simulink model "LgrstOpenLStateCtrl"  (R2018b)
settings: Solver=FixedStepDiscrete  StartTime=0.0  StopTime=10.0  FixedStep=0.01  RelTol=1e-3
libraries: StateCtrlLib x1
settings Model: Creator=sn2xws  LastModifiedBy=sn2xws
settings DataIOCC: SaveFormat=StructureWithTime
settings OptimizationCC: DefaultParameterBehavior=Inlined  EnhancedBackFolding=on  PassReuseOutputArgsAs=Individual arguments  ZeroExternalMemoryAtStartup=off  ZeroInternalMemoryAtStartup=off  OptimizeBlockOrder=speed  DifferentSizesBufferReuse=on  OptimizationCustomize=off
settings DebuggingCC: ParameterTunabilityLossMsg=error
settings ModelReferenceCC: ModelReferenceNumInstancesAllowed=Single
settings SFSimCC: MATLABDynamicMemAlloc=off
settings RTWCC: SystemTargetFile=autosar.tlc  GenCodeOnly=on  TemplateMakefile=ert_default_tmf  Description=AUTOSAR  GenerateReport=on  IncludeHyperlinkInReport=on  LaunchReport=on  GenerateTraceInfo=on  GenerateTraceReport=on  GenerateTraceReportSl=on  GenerateTraceReportSf=on  GenerateTraceReportEml=on
settings CodeAppCC: ForceParamTrailComments=on  IgnoreCustomStorageClasses=off  OperatorAnnotations=on  SimulinkDataObjDesc=on  SFDataObjDesc=on  InsertBlockDesc=on
settings STFCustomTargetCC: TargetLangStandard=C99 (ISO)  MultiwordLength=256  ParMdlRefBuildCompliant=on  CompOptLevelCompliant=on  IncludeMdlTerminateFcn=off  CombineOutputUpdateFcns=on  SuppressErrorStatus=on  ERTCustomFileBanners=on  SupportNonFinite=off  SupportComplex=off  SupportContinuousTime=off  SupportNonInlinedSFcns=off  RemoveResetFunc=on  MATLABClassNameForMDSCustomization=Simulink.SoftwareTarget.ERTCustomization  AutosarCompliant=on  UseToolchainInfoCompliant=on  LookupTableObjectStructAxisOrder=2,1,3,4,...  LUTObjectStructOrderEvenSpacing=Size,Table,Breakpoints  SystemTargetFile=autosar.tlc
settings ERTTargetCC: TargetLangStandard=C99 (ISO)  ConcurrentExecutionCompliant=off  IncludeMdlTerminateFcn=off  SuppressErrorStatus=on  SupportNonFinite=off  SupportComplex=off  ModelStepFunctionPrototypeControlCompliant=off  CPPClassGenCompliant=off  AutosarCompliant=on  LookupTableObjectStructAxisOrder=2,1,3,4,...  LUTObjectStructOrderEvenSpacing=Size,Table,Breakpoints  InlinedParameterPlacement=NonHierarchical  ERTCustomFileTemplate=example_file_process.tlc

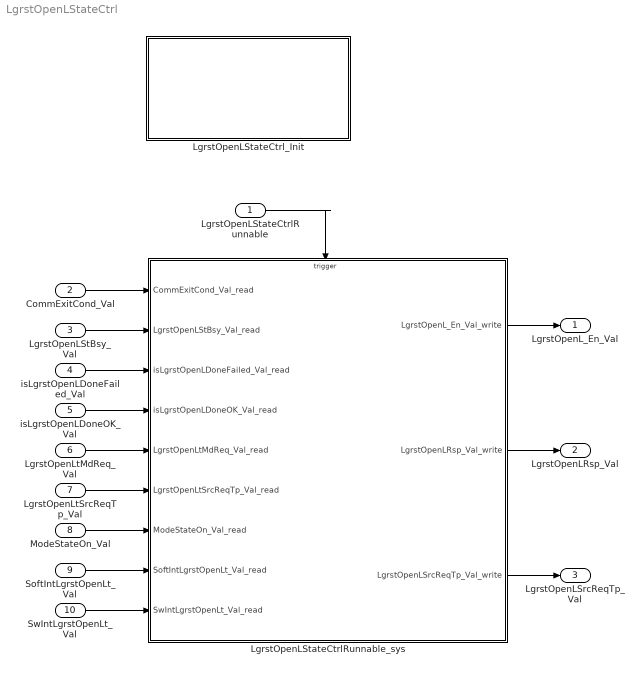
== system LgrstOpenLStateCtrl ==
  LgrstOpenLStateCtrlRunnable : Inport  SampleTime=0.01  OutputFunctionCall=on
  CommExitCond_Val : Inport  Port=2  OutDataTypeStr=boolean  PortDimensions=1
  LgrstOpenLStBsy_Val : Inport  Port=3  OutDataTypeStr=boolean  PortDimensions=1
  isLgrstOpenLDoneFailed_Val : Inport  Port=4  OutDataTypeStr=boolean  PortDimensions=1
  isLgrstOpenLDoneOK_Val : Inport  Port=5  OutDataTypeStr=boolean  PortDimensions=1
  LgrstOpenLtMdReq_Val : Inport  Port=6  OutDataTypeStr=boolean  PortDimensions=1
  LgrstOpenLtSrcReqTp_Val : Inport  Port=7  OutDataTypeStr=Enum: SrcReqTp1  PortDimensions=1
  ModeStateOn_Val : Inport  Port=8  OutDataTypeStr=boolean  PortDimensions=1
  SoftIntLgrstOpenLt_Val : Inport  Port=9  OutDataTypeStr=IntEnable  PortDimensions=1
  SwIntLgrstOpenLt_Val : Inport  Port=10  OutDataTypeStr=IntEnable  PortDimensions=1
  LgrstOpenLStateCtrlRunnable_sys : Subsystem
  LgrstOpenLStateCtrl_Init : Subsystem
  LgrstOpenL_En_Val : Outport  OutDataTypeStr=boolean  PortDimensions=1
  LgrstOpenLRsp_Val : Outport  Port=2  OutDataTypeStr=Enum: MdRspLocal1  PortDimensions=1
  LgrstOpenLSrcReqTp_Val : Outport  Port=3  OutDataTypeStr=Enum: SrcReqTp1  PortDimensions=1
  wires:
  CommExitCond_Val/1 -> LgrstOpenLStateCtrlRunnable_sys/1(CommExitCond_Val_read)
  LgrstOpenLStBsy_Val/1 -> LgrstOpenLStateCtrlRunnable_sys/2(LgrstOpenLStBsy_Val_read)
  isLgrstOpenLDoneFailed_Val/1 -> LgrstOpenLStateCtrlRunnable_sys/3(isLgrstOpenLDoneFailed_Val_read)
  isLgrstOpenLDoneOK_Val/1 -> LgrstOpenLStateCtrlRunnable_sys/4(isLgrstOpenLDoneOK_Val_read)
  LgrstOpenLtMdReq_Val/1 -> LgrstOpenLStateCtrlRunnable_sys/5(LgrstOpenLtMdReq_Val_read)
  LgrstOpenLtSrcReqTp_Val/1 -> LgrstOpenLStateCtrlRunnable_sys/6(LgrstOpenLtSrcReqTp_Val_read)
  ModeStateOn_Val/1 -> LgrstOpenLStateCtrlRunnable_sys/7(ModeStateOn_Val_read)
  SoftIntLgrstOpenLt_Val/1 -> LgrstOpenLStateCtrlRunnable_sys/8(SoftIntLgrstOpenLt_Val_read)
  SwIntLgrstOpenLt_Val/1 -> LgrstOpenLStateCtrlRunnable_sys/9(SwIntLgrstOpenLt_Val_read)
  LgrstOpenLStateCtrlRunnable_sys/1(LgrstOpenL_En_Val_write) -> LgrstOpenL_En_Val/1
  LgrstOpenLStateCtrlRunnable_sys/2(LgrstOpenLRsp_Val_write) -> LgrstOpenLRsp_Val/1
  LgrstOpenLStateCtrlRunnable_sys/3(LgrstOpenLSrcReqTp_Val_write) -> LgrstOpenLSrcReqTp_Val/1
  LgrstOpenLStateCtrlRunnable/1 -> LgrstOpenLStateCtrlRunnable_sys/Trigger

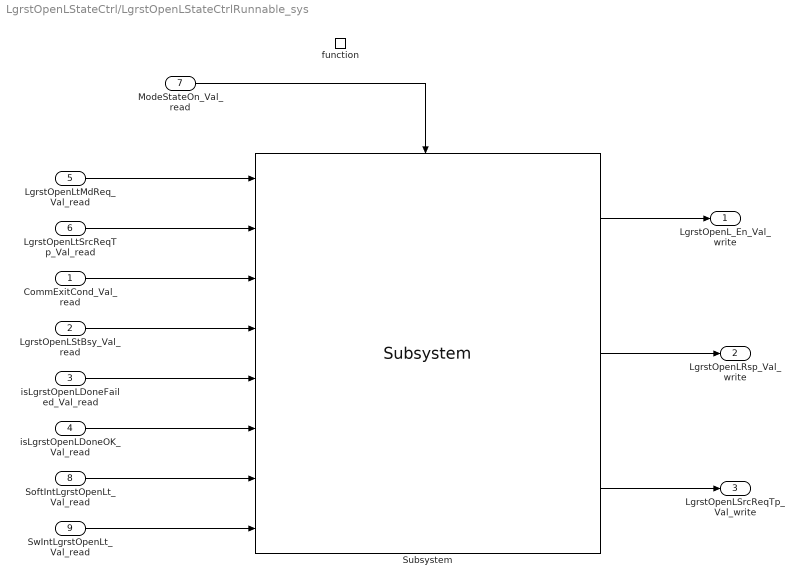
== system LgrstOpenLStateCtrl/LgrstOpenLStateCtrlRunnable_sys ==
  CommExitCond_Val_read : Inport
  LgrstOpenLStBsy_Val_read : Inport  Port=2
  isLgrstOpenLDoneFailed_Val_read : Inport  Port=3
  isLgrstOpenLDoneOK_Val_read : Inport  Port=4
  LgrstOpenLtMdReq_Val_read : Inport  Port=5
  LgrstOpenLtSrcReqTp_Val_read : Inport  Port=6
  ModeStateOn_Val_read : Inport  Port=7
  SoftIntLgrstOpenLt_Val_read : Inport  Port=8
  SwIntLgrstOpenLt_Val_read : Inport  Port=9
  function : TriggerPort  TriggerType=function-call  VariantControl=(inherit)  SampleTimeType=periodic  SampleTime=-1
  Subsystem : StateCtrlLib/Subsystem  SystemSampleTime=-1
  LgrstOpenL_En_Val_write : Outport
      settings: EnsureOutportIsVirtual=on
  LgrstOpenLRsp_Val_write : Outport  Port=2
      settings: EnsureOutportIsVirtual=on
  LgrstOpenLSrcReqTp_Val_write : Outport  Port=3
      settings: EnsureOutportIsVirtual=on
  wires:
  ModeStateOn_Val_read/1 -> Subsystem/Enable
  Subsystem/2 -> LgrstOpenLRsp_Val_write/1
  Subsystem/3 -> LgrstOpenLSrcReqTp_Val_write/1
  Subsystem/1 -> LgrstOpenL_En_Val_write/1
  LgrstOpenLtMdReq_Val_read/1 -> Subsystem/1
  CommExitCond_Val_read/1 -> Subsystem/3
  LgrstOpenLtSrcReqTp_Val_read/1 -> Subsystem/2
  LgrstOpenLStBsy_Val_read/1 -> Subsystem/4
  SoftIntLgrstOpenLt_Val_read/1 -> Subsystem/7
  isLgrstOpenLDoneFailed_Val_read/1 -> Subsystem/5
  SwIntLgrstOpenLt_Val_read/1 -> Subsystem/8
  isLgrstOpenLDoneOK_Val_read/1 -> Subsystem/6

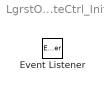
== system LgrstOpenLStateCtrl/LgrstOpenLStateCtrl_Init ==
  Event Listener : EventListener  EventName=reset
